simulink model "projectb"  (R2024a)
settings: Solver=VariableStepAuto  StartTime=0.0  StopTime=10  RelTol=1e-3
undefined symbols (not defined in the file): A, B, C, D, K, L
libraries: slpidlib x1
settings Model: Creator=lostinhaze  LastModifiedBy=lostinhaze

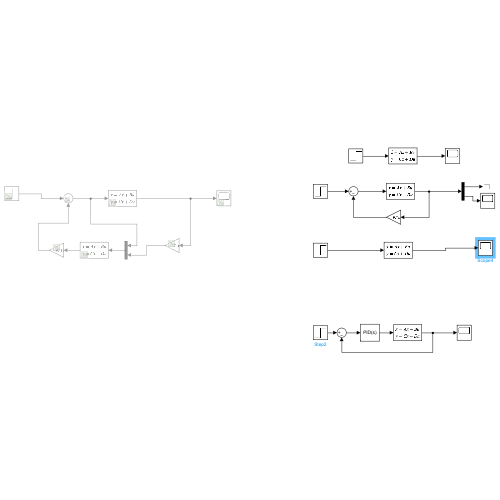
[thumbnail: Simulink's stored preview of the top-level diagram]
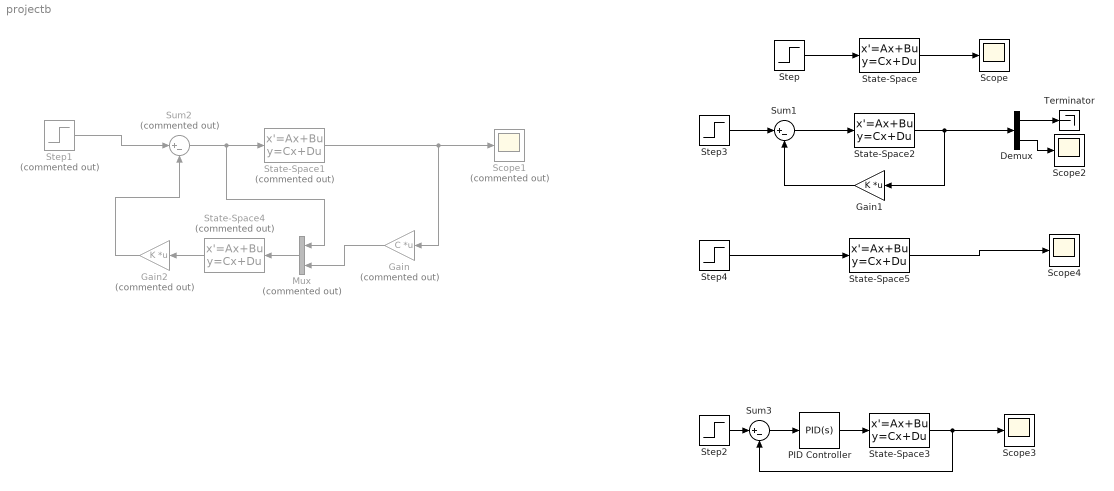
== system projectb ==
  Demux : Demux  Outputs=2
  Gain : Gain  Commented=on  Gain=C  Multiplication=Matrix(K*u)
  Gain1 : Gain  Gain=K  Multiplication=Matrix(K*u)
  Gain2 : Gain  Commented=on  Gain=K  Multiplication=Matrix(K*u)
  Mux : Mux  Commented=on  Inputs=2
  PID Controller : slpidlib/PID Controller  Controller=PID  Form=Parallel  TimeDomain=Continuous-time  UseExternalTs=off  SampleTime=-1  IntegratorMethod=Forward Euler  FilterMethod=Forward Euler  ControllerParametersSource=internal  P=-0.0413903472119066  I=-0.000341909327706851  UseKiTs=off  D=-1.11328962407025  UseExternalDerivativeSource=off  N=161.819781832448  UseFilter=on  TunerSelectOption=Transfer Function Based (PID Tuner App)  InitialConditionSource=internal  InitialConditionForIntegrator=0  InitialConditionForFilter=0  DifferentiatorICPrevScaledInput=0  ExternalReset=none  TrackingMode=off  Kt=1  LimitOutput=off  SatLimitsSource=internal  UpperSaturationLimit=inf  LowerSaturationLimit=-inf  LinearizeAsGain=on  AntiWindupMode=none  Kb=1  LimitIntegrator=off  UpperIntegratorSaturationLimit=inf  LowerIntegratorSaturationLimit=-inf  POutMin=[]  POutMax=[]  IOutMin=[]  IOutMax=[]  DOutMin=[]  DOutMax=[]  NOutMin=[]  NOutMax=[]  SumOutMin=[]  SumOutMax=[]  SaturationOutMin=[]  SaturationOutMax=[]  PParamMin=[]  PParamMax=[]  IParamMin=[]  IParamMax=[]  DParamMin=[]  DParamMax=[]  NParamMin=[]  NParamMax=[]  KbParamMin=[]  KbParamMax=[]  KtParamMin=[]  KtParamMax=[]  KbOutMin=[]  KbOutMax=[]  KtOutMin=[]  KtOutMax=[]  IntegratorOutMin=[]  IntegratorOutMax=[]  FilterOutMin=[]  FilterOutMax=[]  SumI1OutMin=[]  SumI1OutMax=[]  SumI2OutMin=[]  SumI2OutMax=[]  SumI3OutMin=[]  SumI3OutMax=[]  SumI4OutMin=[]  SumI4OutMax=[]  SumDOutMin=[]  SumDOutMax=[]  DifferentiatorOutMin=[]  DifferentiatorOutMax=[]  FilterDiffOutCoefMin=[]  FilterDiffOutCoefMax=[]  ReciprocalOutMin=[]  ReciprocalOutMax=[]  SumDenOutMin=[]  SumDenOutMax=[]  SumNumOutMin=[]  SumNumOutMax=[]  DivideOutMin=[]  DivideOutMax=[]  UdiffTsProdOutMin=[]  UdiffTsProdOutMax=[]  NTsProdOutMin=[]  NTsProdOutMax=[]  UintegralTsProdOutMin=[]  UintegralTsProdOutMax=[]  UngainTsProdOutMin=[]  UngainTsProdOutMax=[]  ClampingZeroOutDataTypeStr=Inherit: Inherit via back propagation  ClampingZeroOutMin=[]  ClampingZeroOutMax=[]  FilterDenConstantOutDataTypeStr=Inherit: Inherit via back propagation  FilterDenConstantOutMin=[]  FilterDenConstantOutMax=[]  PCopyOutDataTypeStr=Inherit: Inherit via back propagation  PCopyOutMin=[]  PCopyOutMax=[]  NCopyOutDataTypeStr=Inherit: Inherit via back propagation  NCopyOutMin=[]  NCopyOutMax=[]  IntegratorContinuousStateAttributes=''  IntegratorStateMustResolveToSignalObject=off  IntegratorRTWStateStorageClass=Auto  FilterContinuousStateAttributes=''  FilterStateMustResolveToSignalObject=off  FilterRTWStateStorageClass=Auto  ParallelPVariant=InternalParameters  IdealPVariant=Disabled  IVariant=InternalParameters  DVariant=InternalParameters  IntegratorVariant=Continuous  SatVariant=Disabled  AWVariant=Passthrough  PCopyVariant=Disabled  TRVariant=Disabled  FdbkBlocksVariant=Forward  IdealPFdbkVariant=Disabled  SatFdbkVariant=Disabled  DerivativeFilterVariant=ContFilter  NVariant=InternalParameters  NCopyVariant=Disabled  FilterICVariant=InternalICsFilter  IntegratorICVariant=InternalICs  ExternalResetVariant=Disabled  TRSumVariant=Passthrough  SumFdbkVariant=Disabled  SumVariant=Sum_PID  TsampFilterVariant=InternalTs  TsampNgainVariant=Passthrough  TsampIntegralVariant=Disabled_SignalSpec  ExternalSaturationOutDataTypeStr=Inherit: Same as second input  DerivativeSourceVariant=ErrorSignal
  Scope{,2..4} (4 alike) : Scope
  Scope1 : Scope  Commented=on
  State-Space : StateSpace  A=[ 0,1,0,0; 0,-0.818,2.6727,0; 0,0,0,1;0,-0.4545,31.1818,0]  B=[0;1.8182;0;4.5455]  C=[1 0 0 0]  D=0  InitialCondition=0
  State-Space1 : StateSpace  Commented=on  A=A  B=B  C=eye(4)  D=[0;0;0;0]  InitialCondition=0
  State-Space2 : StateSpace  A=A  B=B  C=eye(4,4)  D=[0;0;0;0]  InitialCondition=0
  State-Space3 : StateSpace  A=A  B=B  C=C  D=0  InitialCondition=0
  State-Space4 : StateSpace  Commented=on  A=A  B=B  C=eye(4)  D=[0;0;0;0]  InitialCondition=0
  State-Space5 : StateSpace  A=A-L*C  B=B  C=C  D=D  InitialCondition=0
  Step{,2..4} (4 alike) : Step  SampleTime=0
  Step1 : Step  Commented=on  SampleTime=0
  Sum1 : Sum  Inputs=|+-
  Sum2 : Sum  Commented=on  Inputs=|+-
  Sum3 : Sum  Inputs=|+-
  Terminator : Terminator
  wires:
  Step/1 -> State-Space/1
  State-Space/1 -> Scope/1
  Sum1/1 -> State-Space2/1
  Step3/1 -> Sum1/1
  Gain1/1 -> Sum1/2
  State-Space2/1 -> Gain1/1, Demux/1
  Demux/1 -> Terminator/1
  Demux/2 -> Scope2/1
  Step2/1 -> Sum3/1
  Sum3/1 -> PID Controller/1
  PID Controller/1 -> State-Space3/1
  State-Space3/1 -> Sum3/2, Scope3/1
  Gain2/1 -> Sum2/2
  State-Space4/1 -> Gain2/1
  Gain/1 -> Mux/2
  Step1/1 -> Sum2/1
  Mux/1 -> State-Space4/1
  State-Space1/1 -> Gain/1, Scope1/1
  Sum2/1 -> State-Space1/1, Mux/1
  Step4/1 -> State-Space5/1
  State-Space5/1 -> Scope4/1
